simulink model "SIFT-Sysgen"  (R2013a)
settings: Solver=FixedStepDiscrete  SolverMode=SingleTasking  StartTime=0.0  StopTime=10.0  RelTol=1e-3
libraries: xbsIndex_r4 x365, xrbsImage_r4 x64
(part 6 of 10)

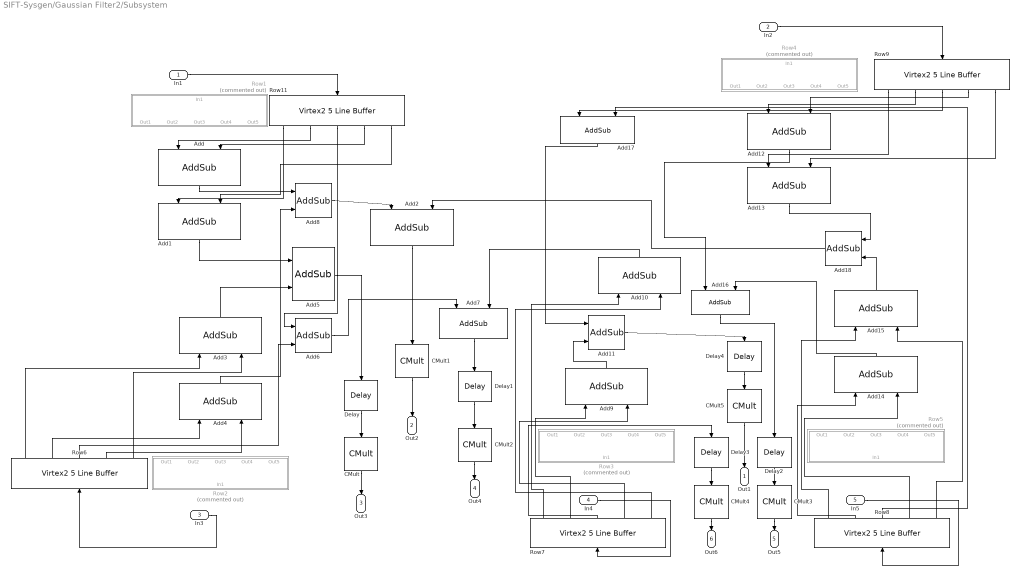
== system SIFT-Sysgen/Gaussian Filter2/Subsystem ==
  In1 : Inport
  In2 : Inport  Port=2
  In3 : Inport  Port=3
  In4 : Inport  Port=4
  In5 : Inport  Port=5
  Add{,1..18} (19 alike) : xbsIndex_r4/AddSub  mode=Addition  use_carryin=off  use_carryout=off  en=off  latency=0  precision=Full  arith_type=Unsigned  n_bits=16  bin_pt=14  quantization=Truncate  overflow=Wrap  dbl_ovrd=off  use_behavioral_HDL=off  hw_selection=Fabric  pipelined=off  block_type=addsub
  CMult : xbsIndex_r4/CMult  const=4  gui_display_data_type=Fixed-point  const_n_bits=8  const_bin_pt=0  float_type=Single  exp_bits=8  fraction_bits=24  en=off  latency=0  precision=Full  arith_type="Signed  (2's comp)"  n_bits=16  bin_pt=14  quantization=Truncate  overflow=Wrap  dbl_ovrd=off  use_behavioral_HDL=off  mem_type=Distributed RAM  pipeline=off  block_type=cmult
  CMult1 : xbsIndex_r4/CMult  const=4  gui_display_data_type=Fixed-point  const_n_bits=8  const_bin_pt=0  float_type=Single  exp_bits=8  fraction_bits=24  en=off  latency=0  precision=Full  arith_type="Signed  (2's comp)"  n_bits=16  bin_pt=14  quantization=Truncate  overflow=Wrap  dbl_ovrd=off  use_behavioral_HDL=off  mem_type=Distributed RAM  pipeline=off  block_type=cmult
  CMult2 : xbsIndex_r4/CMult  const=6  gui_display_data_type=Fixed-point  const_n_bits=8  const_bin_pt=0  float_type=Single  exp_bits=8  fraction_bits=24  en=off  latency=0  precision=Full  arith_type="Signed  (2's comp)"  n_bits=16  bin_pt=14  quantization=Truncate  overflow=Wrap  dbl_ovrd=off  use_behavioral_HDL=off  mem_type=Distributed RAM  pipeline=off  block_type=cmult
  CMult3 : xbsIndex_r4/CMult  const=16  gui_display_data_type=Fixed-point  const_n_bits=8  const_bin_pt=0  float_type=Single  exp_bits=8  fraction_bits=24  en=off  latency=0  precision=Full  arith_type="Signed  (2's comp)"  n_bits=16  bin_pt=14  quantization=Truncate  overflow=Wrap  dbl_ovrd=off  use_behavioral_HDL=off  mem_type=Distributed RAM  pipeline=off  block_type=cmult
  CMult4 : xbsIndex_r4/CMult  const=36  gui_display_data_type=Fixed-point  const_n_bits=8  const_bin_pt=0  float_type=Single  exp_bits=8  fraction_bits=24  en=off  latency=0  precision=Full  arith_type="Signed  (2's comp)"  n_bits=16  bin_pt=14  quantization=Truncate  overflow=Wrap  dbl_ovrd=off  use_behavioral_HDL=off  mem_type=Distributed RAM  pipeline=off  block_type=cmult
  CMult5 : xbsIndex_r4/CMult  const=24  gui_display_data_type=Fixed-point  const_n_bits=8  const_bin_pt=0  float_type=Single  exp_bits=8  fraction_bits=24  en=off  latency=0  precision=Full  arith_type="Signed  (2's comp)"  n_bits=16  bin_pt=14  quantization=Truncate  overflow=Wrap  dbl_ovrd=off  use_behavioral_HDL=off  mem_type=Distributed RAM  pipeline=off  block_type=cmult
  Delay{,1..4} (5 alike) : xbsIndex_r4/Delay  rst=off  infoeditControl=Selection of Reset will increase slice count due to use of real FFs and instead of SRLs  en=off  latency=1  dbl_ovrd=off  reg_retiming=off  block_type=delay
  Row1 : Subsystem  Commented=on
  Row{6..9,11} (5 alike) : xrbsImage_r4/Virtex2 5 Line Buffer  line_size=720  cst=1
      link override Virtex2 Line Buffer/Single Port RAM: block_version=8.2
      link override Virtex2 Line Buffer1/Single Port RAM: block_version=8.2
      link override Virtex2 Line Buffer2/Single Port RAM: block_version=8.2
      link override Virtex2 Line Buffer3/Single Port RAM: block_version=8.2
  Row2 : Subsystem  Commented=on
  Row3 : Subsystem  Commented=on
  Row4 : Subsystem  Commented=on
  Row5 : Subsystem  Commented=on
  Out1 : Outport
  Out2 : Outport  Port=2
  Out3 : Outport  Port=3
  Out4 : Outport  Port=4
  Out5 : Outport  Port=5
  Out6 : Outport  Port=6
  wires:
  In1/1 -> Row11/1
  Row11/2 -> Add/1
  Row11/4 -> Add/2
  Row11/1 -> Add1/1
  Row11/5 -> Add1/2
  Add/1 -> Add8/1
  In3/1 -> Row6/1
  Row6/2 -> Add4/1
  Row6/4 -> Add4/2
  Row6/1 -> Add3/1
  Row6/5 -> Add3/2
  Row6/3 -> Add6/2
  Add4/1 -> Add8/2
  Add3/1 -> Add5/2
  Add1/1 -> Add5/1
  Row11/3 -> Add6/1
  Delay/1 -> CMult/1
  CMult/1 -> Out3/1
  Add5/1 -> Delay/1
  Add8/1 -> Add2/1
  Add2/1 -> CMult1/1
  CMult1/1 -> Out2/1
  Add6/1 -> Add7/1
  Add7/1 -> Delay1/1
  Delay1/1 -> CMult2/1
  CMult2/1 -> Out4/1
  In4/1 -> Row7/1
  Row7/2 -> Add9/1
  Row7/4 -> Add9/2
  Add10/1 -> Add7/2
  Add9/1 -> Add11/2
  Row7/1 -> Add10/1
  Row7/5 -> Add10/2
  Row9/2 -> Add12/1
  Row9/4 -> Add12/2
  Row9/1 -> Add13/1
  Row9/5 -> Add13/2
  Row8/2 -> Add14/1
  Row8/4 -> Add14/2
  Row8/1 -> Add15/1
  Row8/5 -> Add15/2
  In5/1 -> Row8/1
  In2/1 -> Row9/1
  Delay3/1 -> CMult4/1
  Delay2/1 -> CMult3/1
  CMult4/1 -> Out6/1
  CMult3/1 -> Out5/1
  CMult5/1 -> Out1/1
  Delay4/1 -> CMult5/1
  Row7/3 -> Delay3/1
  Add11/1 -> Delay4/1
  Add16/1 -> Delay2/1
  Row9/3 -> Add17/1
  Row8/3 -> Add17/2
  Add14/1 -> Add16/2
  Add15/1 -> Add18/2
  Add13/1 -> Add18/1
  Add12/1 -> Add16/1
  Add17/1 -> Add11/1
  Add18/1 -> Add2/2
